simulink model "ex4improver16"  (R2025b)
settings: Solver=VariableStepAuto  StartTime=0.0  StopTime=280  RelTol=1e-3
values from neighbouring files (symbols this model uses):
  K = nmpc_design_st2(par)    [ex4.m]
  ref = [0;0]    [ex4.m]
settings Model: Creator=Esteban  LastModifiedBy=Esteban

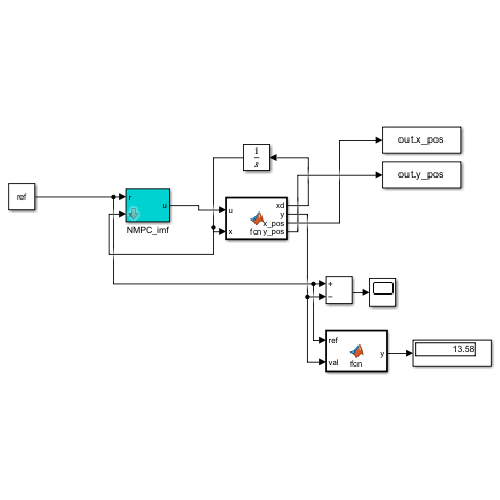
[thumbnail: Simulink's stored preview of the top-level diagram]
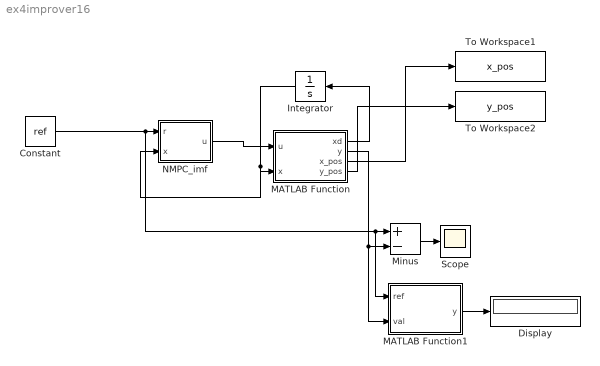
== system ex4improver16 ==
  Constant : Constant  Value=ref
  Display : Display
  Integrator : Integrator  InitialCondition=[-3000;600;0]
  MATLAB Function : MATLAB Function  TreatAsAtomicUnit=on
  MATLAB Function1 : MATLAB Function  TreatAsAtomicUnit=on
  Minus : Sum  Inputs=+-
  NMPC_imf : Subsystem  mask{K=K}
      mask prompts: K "NMPC structure"
  Scope : Scope
      settings: ActiveDisplayYMinimum=-441.09311963052926  ActiveDisplayYMaximum=1129.3369559500566
  To Workspace1 : ToWorkspace  VariableName=x_pos  SaveFormat=Timeseries  SampleTime=-1
  To Workspace2 : ToWorkspace  VariableName=y_pos  SaveFormat=Timeseries  SampleTime=-1
  wires:
  MATLAB Function/1(xd) -> Integrator/1
  Integrator/1 -> NMPC_imf/2(x), MATLAB Function/2(x)
  NMPC_imf/1(u) -> MATLAB Function/1(u)
  Constant/1 -> MATLAB Function1/1(ref), Minus/1, NMPC_imf/1(r)
  MATLAB Function/2(y) -> MATLAB Function1/2(val), Minus/2
  Minus/1 -> Scope/1
  MATLAB Function1/1(y) -> Display/1
  MATLAB Function/3(x_pos) -> To Workspace1/1
  MATLAB Function/4(y_pos) -> To Workspace2/1

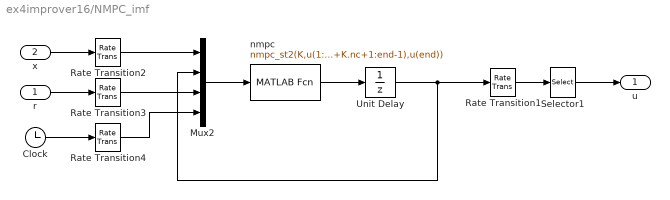
== system ex4improver16/NMPC_imf ==
  r : Inport
  x : Inport  Port=2
  Clock : Clock
  Mux2 : Mux
  Rate Transition{1..4} (4 alike) : RateTransition  OutPortSampleTime=K.Ts
  Selector1 : Selector  InputPortWidth=K.nc  IndexOptions=Index vector (dialog)  Indices=1:K.nu  OutputSizes=1
  Unit Delay : UnitDelay  InitialCondition=zeros(K.nc,1)  SampleTime=K.Ts  HasFrameUpgradeWarning=on
  nmpc : MATLABFcn  MATLABFcn=nmpc_st2(K,u(1:K.nx),u(K.nx+1:K.nx+K.nc),u(K.nx+K.nc+1:end-1),u(end))  OutputDimensions=K.nc
  u : Outport  PortDimensions=K.nu
  wires:
  x/1 -> Rate Transition2/1
  Unit Delay/1 -> Rate Transition1/1, Mux2/2
  Mux2/1 -> nmpc/1
  r/1 -> Rate Transition3/1
  Rate Transition2/1 -> Mux2/1
  Rate Transition1/1 -> Selector1/1
  Rate Transition3/1 -> Mux2/3
  nmpc/1 -> Unit Delay/1
  Selector1/1 -> u/1
  Clock/1 -> Rate Transition4/1
  Rate Transition4/1 -> Mux2/4

== matlab function ex4improver16/MATLAB Function1 ==
  data: ref input; y output; val input
function y = fcn(ref,val)

y = norm(ref-val);

== matlab function ex4improver16/MATLAB Function ==
  data: xd output; u input; y output; x input; x_pos output; y_pos output
function [xd,y,x_pos,y_pos] = fcn(u,x)
l = 1.5;
th = x(3,:);
xd = [u(1)*cos(th);
     u(1)*sin(th);
     u(1)/l*tan(u(2))];
y = [x(1);x(2)];

x_pos = x(1);
y_pos = x(2);
